simulink model "ex5modelo"  (R2017a)
settings: Solver=VariableStepAuto  StartTime=0.0  StopTime=20  RelTol=1e-3
settings Model: Creator=asm  LastModifiedBy=asm

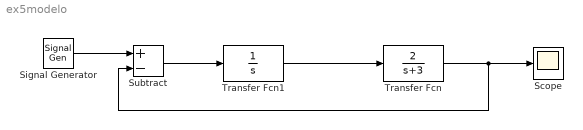
== system ex5modelo ==
  Scope : Scope
  Signal Generator : SignalGenerator  WaveForm=square  Frequency=0.3  Units=rad/sec
  Subtract : Sum  Inputs=+-
  Transfer Fcn : TransferFcn  Numerator=[2]  Denominator=[1 3]
  Transfer Fcn1 : TransferFcn  Denominator=[1 0]
  wires:
  Signal Generator/1 -> Subtract/1
  Transfer Fcn/1 -> Subtract/2, Scope/1
  Subtract/1 -> Transfer Fcn1/1
  Transfer Fcn1/1 -> Transfer Fcn/1
